simulink model "controltest"  (Simulink 7.9)
settings: Solver=ode45  StartTime=0.0  StopTime=5  MaxStep=0.001  RelTol=1e-3
settings Model: Creator=naa  LastModifiedBy=k340h17

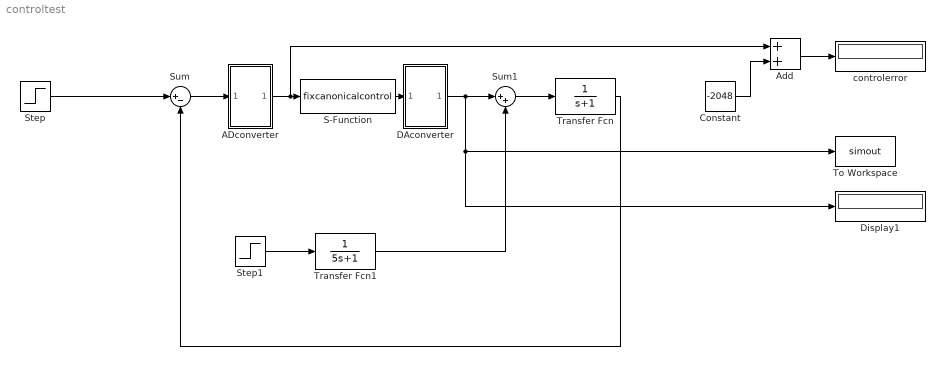
== system controltest ==
  ADconverter : Subsystem  mask{Vinmin=-1, Vinmax=1, ADoutmin=0, ADoutmax=32767, Tsample=0.01}
      mask prompts: Vinmin "Vin min"; Vinmax "Vin max"; ADoutmin "ADout min"; ADoutmax "ADout max"; Tsample "Sampletime"
  Add : Sum
  Constant : Constant  Value=-2048
  DAconverter : Subsystem  mask{Voutmin=-1, Voutmax=1, DAinmin=0, DAinmax=32768, Tsample=0.01}
      mask prompts: Voutmin "Vout min"; Voutmax "Vout max"; DAinmin "DAin min"; DAinmax "DAin max"; Tsample "Sampletime"
  Display1 : Display
  S-Function : S-Function  FunctionName=fixcanonicalcontrol  Parameters=32768 16385 2 307109 1 0 32767  EnableBusSupport=off
  Step : Step  Time=0.1  After=3  SampleTime=0
  Step1 : Step  Time=0.1  After=0  SampleTime=0
  Sum : Sum  Inputs=|+-
  Sum1 : Sum  Inputs=|++
  To Workspace : ToWorkspace  VariableName=simout  SampleTime=-1  SaveFormat=Timeseries
  Transfer Fcn : TransferFcn  Denominator=[1 1]
  Transfer Fcn1 : TransferFcn  Denominator=[5 1]
  controlerror : Display
  wires:
  Sum/1 -> ADconverter/1(In1)
  Sum1/1 -> Transfer Fcn/1
  Step1/1 -> Transfer Fcn1/1
  Transfer Fcn1/1 -> Sum1/2
  ADconverter/1(Out1) -> S-Function/1, Add/1
  S-Function/1 -> DAconverter/1(In1)
  Add/1 -> controlerror/1
  Constant/1 -> Add/2
  DAconverter/1(Out1) -> Sum1/1, Display1/1, To Workspace/1
  Transfer Fcn/1 -> Sum/2
  Step/1 -> Sum/1

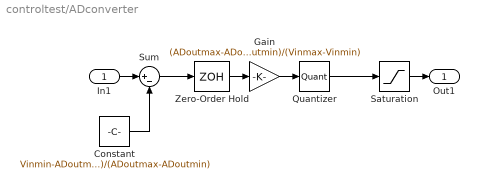
== system controltest/ADconverter ==
  In1 : Inport
  Constant : Constant  Value=Vinmin-ADoutmin*(Vinmax-Vinmin)/(ADoutmax-ADoutmin)
  Gain : Gain  Gain=(ADoutmax-ADoutmin)/(Vinmax-Vinmin)
  Quantizer : Quantizer  QuantizationInterval=1
  Saturation : Saturate  UpperLimit=ADoutmax  LowerLimit=ADoutmin
  Sum : Sum  Inputs=|+-
  Zero-Order Hold : ZeroOrderHold  SampleTime=Tsample
  Out1 : Outport
  wires:
  Quantizer/1 -> Saturation/1
  Constant/1 -> Sum/2
  Gain/1 -> Quantizer/1
  In1/1 -> Sum/1
  Saturation/1 -> Out1/1
  Zero-Order Hold/1 -> Gain/1
  Sum/1 -> Zero-Order Hold/1

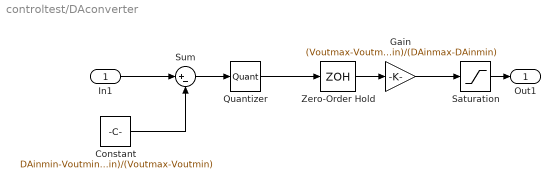
== system controltest/DAconverter ==
  In1 : Inport
  Constant : Constant  Value=DAinmin-Voutmin*(DAinmax-DAinmin)/(Voutmax-Voutmin)
  Gain : Gain  Gain=(Voutmax-Voutmin)/(DAinmax-DAinmin)
  Quantizer : Quantizer  QuantizationInterval=1
  Saturation : Saturate  UpperLimit=Voutmax  LowerLimit=Voutmin
  Sum : Sum  Inputs=|+-
  Zero-Order Hold : ZeroOrderHold  SampleTime=Tsample
  Out1 : Outport
  wires:
  Constant/1 -> Sum/2
  In1/1 -> Sum/1
  Saturation/1 -> Out1/1
  Zero-Order Hold/1 -> Gain/1
  Gain/1 -> Saturation/1
  Quantizer/1 -> Zero-Order Hold/1
  Sum/1 -> Quantizer/1
